simulink model "dc_series_motor_performance_C2000"  (R2017a)
settings: Solver=FixedStepAuto  StartTime=0.0  StopTime=0.6  RelTol=1e-3
libraries: c2802xlib x2
settings Model: Creator=Md Aadil  LastModifiedBy=Md Aadil
settings OptimizationCC: DefaultParameterBehavior=Inlined  UseDivisionForNetSlopeComputation=on  UseFloatMulNetSlope=on  InlineInvariantSignals=on  PassReuseOutputArgsAs=Individual arguments  ZeroExternalMemoryAtStartup=off  ZeroInternalMemoryAtStartup=off  NoFixptDivByZeroProtection=on  EfficientFloat2IntCast=on  LifeSpan=1
settings DebuggingCC: ParameterTunabilityLossMsg=error
settings HardwareCC: ProdBitPerChar=16  ProdBitPerInt=16  ProdBitPerPointer=32  ProdBitPerSizeT=32  ProdBitPerPtrDiffT=32  ProdLargestAtomicInteger=Integer  ProdLargestAtomicFloat=None  ProdWordSize=16  ProdHWDeviceType=Texas Instruments->C2000
settings SFSimCC: MATLABDynamicMemAlloc=off
settings RTWCC: SystemTargetFile=ert.tlc  TemplateMakefile=ert_default_tmf  Description=Embedded Coder  GenerateReport=on  IncludeHyperlinkInReport=on  LaunchReport=on  GenerateTraceInfo=on  GenerateTraceReport=on  GenerateTraceReportSl=on  GenerateTraceReportSf=on  GenerateTraceReportEml=on  GenerateCodeMetricsReport=on
settings CodeAppCC: ForceParamTrailComments=on  IgnoreCustomStorageClasses=off  OperatorAnnotations=on  SimulinkDataObjDesc=on  SFDataObjDesc=on  MATLABFcnDesc=on  CustomSymbolStrGlobalVar=rt$N$M  CustomSymbolStrType=$N$M  CustomSymbolStrFcn=$N$M$F  CustomSymbolStrMacro=$N$M  InsertBlockDesc=on  MATLABSourceComments=on
settings ERTTargetCC: TargetLangStandard=C99 (ISO)  GenerateSampleERTMain=on  IncludeMdlTerminateFcn=off  CombineSignalStateStructs=on  SupportComplex=off  SupportContinuousTime=on  SupportNonInlinedSFcns=on  InlinedParameterPlacement=NonHierarchical  ERTCustomFileTemplate=example_file_process.tlc  ERTFilePackagingFormat=CompactWithDataFile

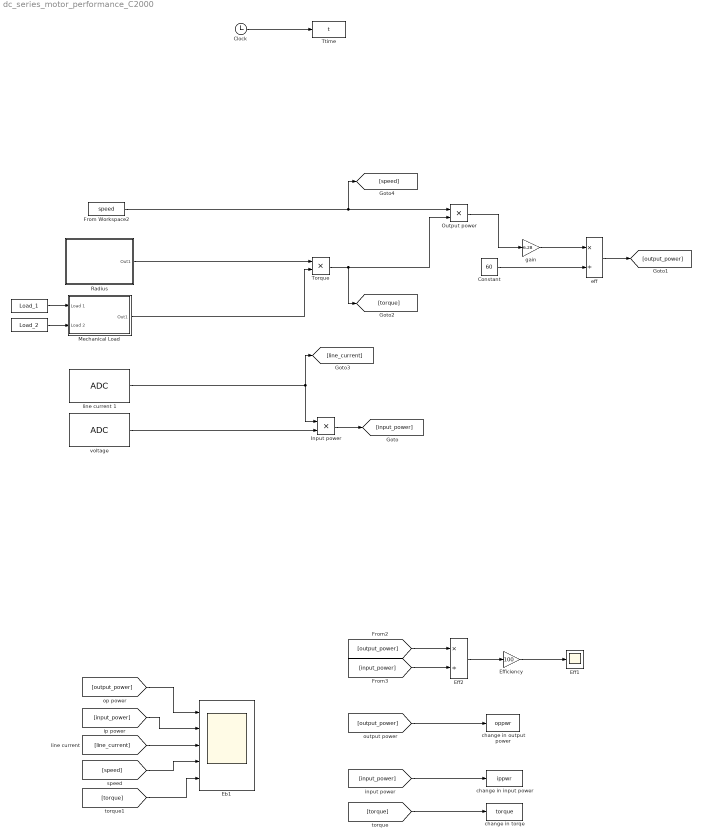
== system dc_series_motor_performance_C2000 ==
  " " : FromWorkspace  VariableName=Load_1
  "  " : FromWorkspace  VariableName=Load_2
  Clock : Clock
  Constant : Constant  Value=60
  Eb1 : Scope  NumInputPorts=5
  "Eff1 " : Scope
  "Eff2 " : Product  Inputs=*/
  "Efficiency " : Gain  Gain=100
  From Workspace2 : FromWorkspace  VariableName=speed  SampleTime=1
  Input power : Product
  Mechanical Load : Subsystem
  Output power : Product
  Radius : Subsystem
  Torque : Product
  Ttime : ToWorkspace  VariableName=t  SampleTime=-1
  "change in input power " : ToWorkspace  VariableName=ippwr  SampleTime=-1
  change in output power : ToWorkspace  VariableName=oppwr  SampleTime=-1
  change in torqe : ToWorkspace  VariableName=torque  SampleTime=-1
  eff : Product  Inputs=*/
  gain : Gain  Gain=6.28
  line current 1 : c2802xlib/ADC  ADCModule=1  samplingMode=Single sample mode  ADCResolution=12-bit (Single-ended input)  useSOC1=SOC2  useSOC2=SOC0_SOC1  SOCAcquisitionWindow=7  SOCTriggerSource=Software  SOCInterruptTrigger=No ADCINT  Ts=0.001  dType=double  postInterrupt=off  interruptSel=ADCINT1  ADCINTContinuous=on  endma=off  chdma=1  blkParamProc=C2000  conv1=ADCINA2  conv2=ADCINA0 and ADCINB0  conv1_Type4=ADCIN0  conv2_Type4=ADCIN0 and ADCIN1
      settings: SourceProductName=Embedded Coder Support Package for Texas Instruments C2000 Processors
  voltage : c2802xlib/ADC  ADCModule=1  samplingMode=Single sample mode  ADCResolution=12-bit (Single-ended input)  useSOC1=SOC1  useSOC2=SOC0_SOC1  SOCAcquisitionWindow=7  SOCTriggerSource=Software  SOCInterruptTrigger=No ADCINT  Ts=0.001  dType=double  postInterrupt=off  interruptSel=ADCINT1  ADCINTContinuous=on  endma=off  chdma=1  blkParamProc=C2000  conv1=ADCINA1  conv2=ADCINA0 and ADCINB0  conv1_Type4=ADCIN0  conv2_Type4=ADCIN0 and ADCIN1
      settings: SourceProductName=Embedded Coder Support Package for Texas Instruments C2000 Processors
  wires:
  [line_current] -> Eb1/3
  [output_power] -> "Eff2 "/1
  [output_power] -> Eb1/1
  [torque] -> change in torqe/1
  [speed] -> Eb1/4
  line current 1/1 -> [line_current], Input power/1
  [output_power] -> change in output power/1
  From Workspace2/1 -> [speed], Output power/1
  "  "/1 -> Mechanical Load/2(Load 2)
  Torque/1 -> [torque], Output power/2
  [input_power] -> "Eff2 "/2
  voltage/1 -> Input power/2
  Radius/1(Out1) -> Torque/1
  [input_power] -> Eb1/2
  [input_power] -> "change in input power "/1
  Mechanical Load/1(Out1) -> Torque/2
  Clock/1 -> Ttime/1
  Input power/1 -> [input_power]
  " "/1 -> Mechanical Load/1(Load 1)
  [torque] -> Eb1/5
  Constant/1 -> eff/2
  eff/1 -> [output_power]
  gain/1 -> eff/1
  Output power/1 -> gain/1
  "Eff2 "/1 -> "Efficiency "/1
  "Efficiency "/1 -> "Eff1 "/1

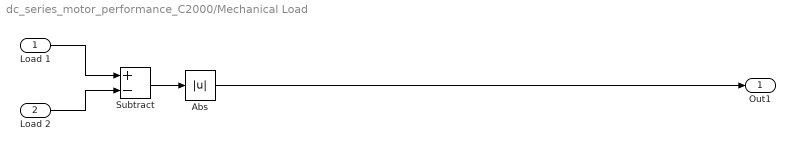
== system dc_series_motor_performance_C2000/Mechanical Load ==
  Load 1 : Inport
  Load 2 : Inport  Port=2
  Abs : Abs
  Subtract : Sum  Inputs=+-
  Out1 : Outport
  wires:
  Load 1/1 -> Subtract/1
  Load 2/1 -> Subtract/2
  Abs/1 -> Out1/1
  Subtract/1 -> Abs/1

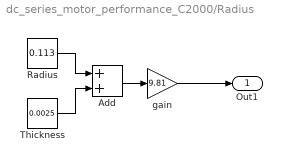
== system dc_series_motor_performance_C2000/Radius ==
  Add : Sum
  Radius : Constant  Value=0.113
  Thickness : Constant  Value=0.0025
  gain : Gain  Gain=9.81
  Out1 : Outport
  wires:
  Radius/1 -> Add/1
  Thickness/1 -> Add/2
  Add/1 -> gain/1
  gain/1 -> Out1/1
